simulink model "Ex3_3_a_sim"  (R2025b)
settings: Solver=ode45  StartTime=0.0  StopTime=0.2  RelTol=1e-3  EnableMultiTasking=on
values from neighbouring files (symbols this model uses):
  D = 1e-5    (= 1e-05)    [Ex3_3_a.m]
  J = 1e-5    (= 1e-05)    [Ex3_3_a.m]
  K_e = 5e-2    (= 0.05)    [Ex3_3_a.m]
  K_t = 5e-2    (= 0.05)    [Ex3_3_a.m]
  L = 1e-3    (= 0.001)    [Ex3_3_a.m]
  R = 5.0    (= 5)    [Ex3_3_a.m]
undefined symbols (not defined in the file or in its folder): t_load
settings Model: Creator=Shin
settings SolverCC: AlgebraicLoopSolver=TrustRegion
settings DataIOCC: LimitDataPoints=on  SaveFormat=Array  ReturnWorkspaceOutputs=off
settings OptimizationCC: LifeSpan=inf
settings DebuggingCC: SolverPrmCheckMsg=warning  UnconnectedInputMsg=warning  UnconnectedOutputMsg=warning  UnconnectedLineMsg=warning  SFUnexpectedBacktrackingDiag=warning  SFNoUnconditionalDefaultTransitionDiag=warning  SFExecutionAtInitializationDiag=none  ArithmeticOperatorsInVariantConditions=warning
settings HardwareCC: ProdBitPerPointer=32.0  ProdBitPerSizeT=32.0  ProdBitPerPtrDiffT=32.0  ProdLargestAtomicFloat=None  ProdIntDivRoundTo=Undefined  ProdEndianess=Unspecified  ProdWordSize=32.0  ProdHWDeviceType=32-bit Generic
settings ModelReferenceCC: EnableRefExpFcnMdlSchedulingChecks=on  PropagateSignalLabelsOutOfModel=off
settings SFSimCC: SimUseLocalCustomCode=off  CustomCodeUndefinedFunction=UseInterfaceOnly
settings RTWCC: RTWUseLocalCustomCode=off  GPUComputeCapability=3.5
settings CodeAppCC: StateflowObjectComments=on
settings GRTTargetCC: TargetLangStandard=C89/C90 (ANSI)
settings ConfigComp: CovMetricSettings=dw  CovSaveCumulativeToWorkspaceVar=on  CovSaveSingleToWorkspaceVar=on  CovExternalEMLEnable=off  CovSFcnEnable=off

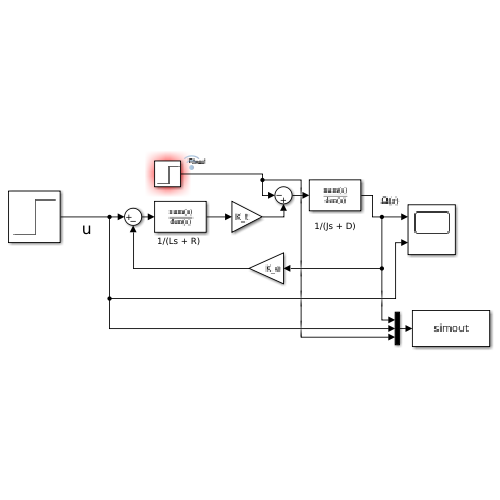
[thumbnail: Simulink's stored preview of the top-level diagram]
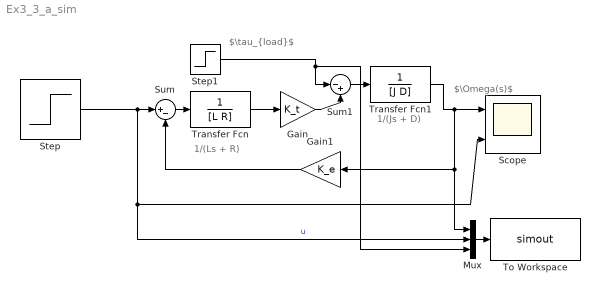
== system Ex3_3_a_sim ==
  note: $\tau_{load}$
  note: $\Omega(s)$
  note: 1/(Js + D)
  note: 1/(Ls + R)
  Gain : Gain  Gain=K_t
  Gain1 : Gain  Gain=K_e
  Mux : Mux  Inputs=3
  Scope : Scope  NumInputPorts=2
      settings: ActiveDisplayYMinimum=-2.45097  ActiveDisplayYMaximum=22.0587  DataLoggingSaveFormat=Array
  Step : Step  Time=0.01  SampleTime=0
  Step1 : Step  Time=0.05  After=t_load  SampleTime=0
  Sum : Sum  Inputs=|+-
  Sum1 : Sum  Inputs=|-+
  To Workspace : ToWorkspace  VariableName=simout  SaveFormat=Timeseries  SampleTime=-1
  Transfer Fcn : TransferFcn  Denominator=[L R]
  Transfer Fcn1 : TransferFcn  Denominator=[J D]
  wires:
  Step/1 -> Sum/1, Mux/2, Scope/2  "u"
  Mux/1 -> To Workspace/1
  Transfer Fcn/1 -> Gain/1
  Sum/1 -> Transfer Fcn/1
  Gain1/1 -> Sum/2
  Transfer Fcn1/1 -> Scope/1, Gain1/1, Mux/1
  Gain/1 -> Sum1/2
  Sum1/1 -> Transfer Fcn1/1
  Step1/1 -> Mux/3, Sum1/1
